simulink model "verification_simulink_simplified"  (R2015a)
settings: Solver=ode3  StartTime=0.0  StopTime=T_sim_length  FixedStep=T_sim  RelTol=1e-3
values from neighbouring files (symbols this model uses):
  Ad = sys_discrete.a + L * C + sys_discrete.b * K    [example_integrator.m]    (also in param_pendulum_calc.m)
  Ap = [0, 1; 0, 0]    [example_integrator.m]    (also in param_pendulum.m = [0, 1; upright * omega0 ^ 2, -2 * xi * omega0])
  Bd = -L    [example_integrator.m]    (also in param_pendulum_calc.m)
  Bp = [0; 1]    [example_integrator.m]    (also in example_mimo.m = [Bp, Bp]; param_pendulum.m = [0; omega0 / 9.81])
  C = [1, 0]    [example_integrator.m]    (also in example_mimo.m = [C; C]; param_pendulum.m)
  Cd = K    [example_integrator.m]    (also in param_pendulum_calc.m)
  delay_u_sim = simulink_struct_from_value_vector(round(delay_u / T_sim, 4))    [example_pendulum_static_delay.m]    (also in verification_compare_timevarying_qoc.m = simulink_struct_from_value_vector(delay_u_sim'))
  delay_y_sim = simulink_struct_from_value_vector(round(delay_y / T_sim, 4))    [example_pendulum_static_delay.m]    (also in verification_compare_timevarying_qoc.m = simulink_struct_from_value_vector(delay_y_sim'))
  Gp = [0; 1]    [example_integrator.m]    (also in param_pendulum.m)
  N_p = 1e-2    (= 0.01)    [example_integrator.m]    (also in example_mimo.m = blkdiag(N_p, N_p) * 2; param_pendulum.m = 1e-06)
  Q_tilde = [0.00968, 0; 0, 0.0470]    [example_integrator.m]    (also in param_pendulum.m = 550 * eye(2))
  R_tilde = 0.768    [example_integrator.m]    (also in example_mimo.m = blkdiag(R_tilde, R_tilde) * 2; param_pendulum.m = 0.8)
  T = 1    [example_integrator.m]    (also in param_pendulum.m = 0.2)
  T_sim = T * 1e-3    (= 0.001)    [example_integrator.m]    (also in param_pendulum.m = 0.0001)
libraries: simulink x1
settings Model: SimulationMode=accelerator  Creator=ak22emur  LastModifiedBy=ak22emur

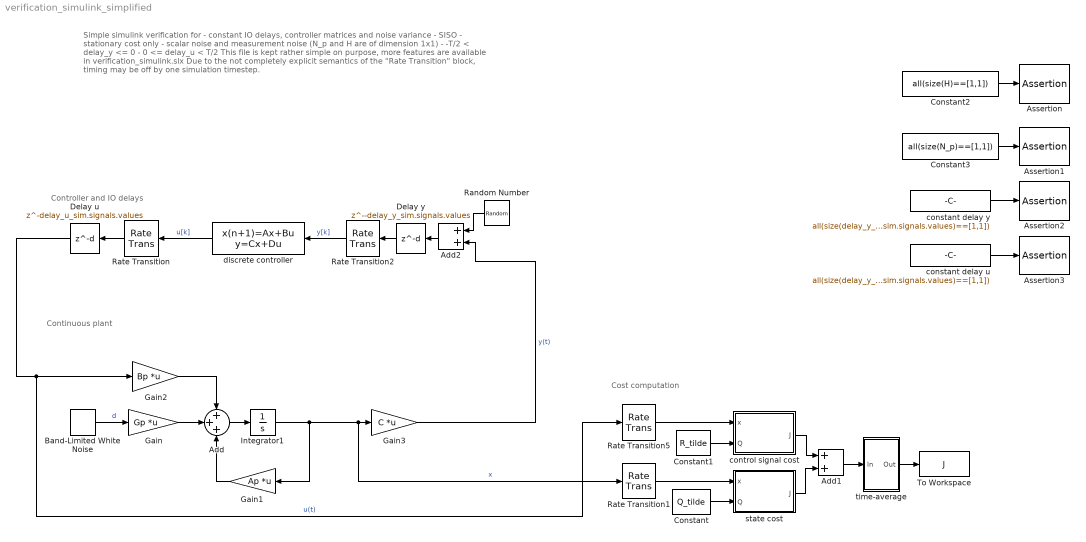
== system verification_simulink_simplified ==
  note: Cost computation
  note: Continuous plant
  note: Controller and IO delays
  note: Simple simulink verification for
      | - constant IO delays, controller matrices and noise variance
      | - SISO
      | - stationary cost only
      | - scalar noise and measurement noise (N_p and H are of dimension 1x1)
      | - -T/2 < delay_y <= 0
      | - 0 <= delay_u < T/2
      |
      | This file is kept rather simple on purpose, more features are available in verification_simulink.slx
      |
      | Due to the not completely explicit semantics of the "Rate Transition" block, timing may be off by one simulation timestep.
  Add : Sum  Inputs=+++
  Add1 : Sum
  Add2 : Sum
  Assertion{,1..3} (4 alike) : Assertion
  Band-Limited White Noise : simulink/Sources/Band-Limited White Noise  Cov=H  Ts=T_sim  seed=[23341]
  Constant : Constant  Value=Q_tilde
  Constant1 : Constant  Value=R_tilde
  Constant2 : Constant  Value=all(size(H)==[1,1])
  Constant3 : Constant  Value=all(size(N_p)==[1,1])
  Delay u : Delay  DelayLength=delay_u_sim.signals.values  DelayLengthUpperLimit=T/T_sim
  Delay y : Delay  DelayLength=-delay_y_sim.signals.values  DelayLengthUpperLimit=T/T_sim
  Gain : Gain  Gain=Gp  Multiplication=Matrix(K*u)
  Gain1 : Gain  Gain=Ap  Multiplication=Matrix(K*u)
  Gain2 : Gain  Gain=Bp  Multiplication=Matrix(K*u)
  Gain3 : Gain  Gain=C  Multiplication=Matrix(K*u)
  Integrator1 : Integrator
  Random Number : RandomNumber  Variance=N_p  Seed=13379812  SampleTime=T_sim
  Rate Transition : RateTransition  Deterministic=off  OutPortSampleTime=0
  Rate Transition1 : RateTransition  OutPortSampleTime=T
  Rate Transition2 : RateTransition  OutPortSampleTime=T
  Rate Transition5 : RateTransition  OutPortSampleTime=T
  To Workspace : ToWorkspace  VariableName=J  SampleTime=-1
      settings: MaxDataPoints=1
  constant delay u : Constant  Value=all(size(delay_y_sim.signals.values)==[1,1])
  constant delay y : Constant  Value=all(size(delay_y_sim.signals.values)==[1,1])
  control signal cost : MATLAB Function  TreatAsAtomicUnit=on
  discrete controller : DiscreteStateSpace  A=Ad  B=Bd  C=Cd  D=0  SampleTime=T
  state cost : MATLAB Function  TreatAsAtomicUnit=on
  time-average : Subsystem
  wires:
  Band-Limited White Noise/1 -> Gain/1  "d"
  Integrator1/1 -> Gain1/1, Rate Transition1/1, Gain3/1  "x"
  Add/1 -> Integrator1/1
  Gain/1 -> Add/2
  Gain1/1 -> Add/3
  Constant/1 -> state cost/2(Q)
  Gain2/1 -> Add/1
  Gain3/1 -> Add2/2  "y(t)"
  Constant1/1 -> control signal cost/2(Q)
  discrete controller/1 -> Rate Transition/1  "u[k]"
  Rate Transition2/1 -> discrete controller/1  "y[k]"
  Rate Transition/1 -> Delay u/1
  Add2/1 -> Delay y/1
  Random Number/1 -> Add2/1
  Rate Transition5/1 -> control signal cost/1(x)
  Add1/1 -> time-average/1(In)
  control signal cost/1(J) -> Add1/1
  state cost/1(J) -> Add1/2
  Rate Transition1/1 -> state cost/1(x)
  time-average/1(Out) -> To Workspace/1
  Constant2/1 -> Assertion/1
  Constant3/1 -> Assertion1/1
  constant delay y/1 -> Assertion2/1
  constant delay u/1 -> Assertion3/1
  Delay u/1 -> Rate Transition5/1, Gain2/1  "u(t)"
  Delay y/1 -> Rate Transition2/1

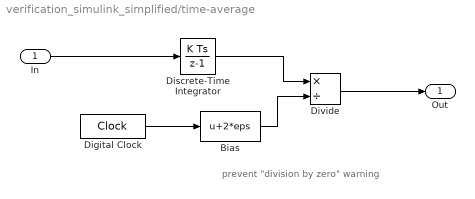
== system verification_simulink_simplified/time-average ==
  note: prevent "division by zero" warning
  In : Inport
  Bias : Bias  Bias=2*eps
  Digital Clock : DigitalClock  SampleTime=T
  Discrete-Time Integrator : DiscreteIntegrator  InitialConditionSetting=State (most efficient)  SampleTime=T
  Divide : Product  Inputs=*/
  Out : Outport
  wires:
  Bias/1 -> Divide/2
  Divide/1 -> Out/1
  Digital Clock/1 -> Bias/1
  Discrete-Time Integrator/1 -> Divide/1
  In/1 -> Discrete-Time Integrator/1

== matlab function verification_simulink_simplified/control signal cost ==
  data: x input; J output; Q input
function J = cost(x,Q)
%#codegen

J=x'*Q*x;

== matlab function verification_simulink_simplified/state cost ==
  data: x input; J output; Q input
function J = cost(x,Q)
%#codegen

J=x'*Q*x;
